simulink model "hps_autopilot_simulink_control_loop"  (R2020a)
settings: Solver=VariableStepAuto  StartTime=0.0  StopTime=10.0  RelTol=1e-3
values from neighbouring files (symbols this model uses):
  Kd = 4    [arduino_matlab.m]
  Ki = 1    [arduino_matlab.m]
  Kp = 1    [arduino_matlab.m]
libraries: checkpacklib x2
settings Model: Creator=ASDFGHJKL  LastModifiedBy=ASDFGHJKL

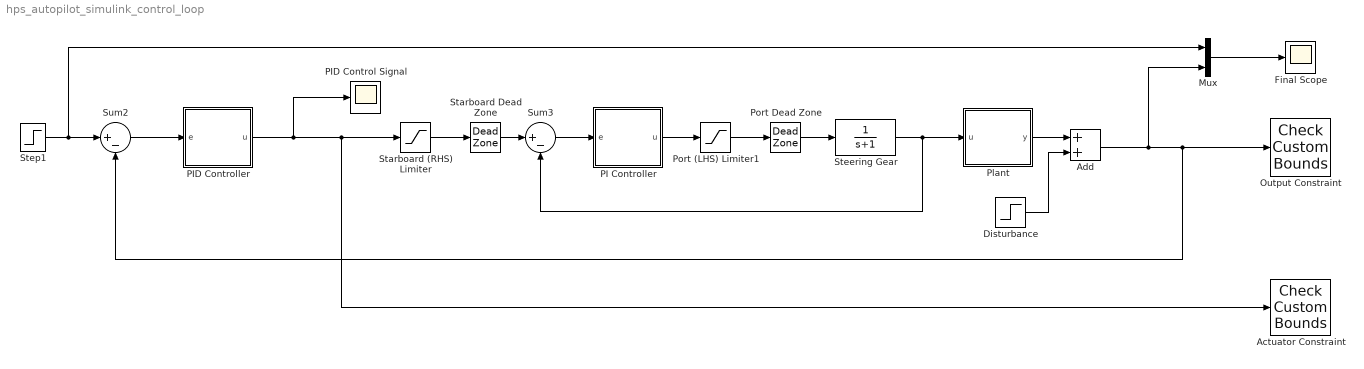
== system hps_autopilot_simulink_control_loop ==
  Actuator Constraint : checkpacklib/Check Custom Bounds  StatePerturbationForJacobian=1.0e-05  InstantiateOnLoad=on  enabled=on  stopWhenAssertionFail=off  export=off  ViewDlgPos=[771.198125 328.725833333334 693.23875 313.738333333334]  OpenViewOnLoad=off  LaunchViewOnOpen=on  TimeUnits=seconds  EnableUpperBound=on  UpperBoundTimes=[0 2.1272365805169;2.1272365805169 20]  UpperBoundAmplitudes=[3.90980563940252 3.90980563940252;0.939113549007046 0.939113549007046]  EnableLowerBound=on  LowerBoundTimes=[0 2.1272365805169;2.1272365805169 20]  LowerBoundAmplitudes=[-3.99363741734438 -3.99363741734438;-0.524055092889176 -0.524055092889176]
      settings: SourceProductBaseCode=CT,ID,MT,SO
  Add : Sum
  Disturbance : Step
  Final Scope : Scope
      settings: StatePerturbationForJacobian=1.0e-05
  Mux : Mux  Inputs=2
  Output Constraint : checkpacklib/Check Custom Bounds  StatePerturbationForJacobian=1.0e-05  InstantiateOnLoad=on  enabled=on  stopWhenAssertionFail=off  export=off  ViewDlgPos=[111.541875 327.726666666666 650.06125 311.74]  OpenViewOnLoad=off  LaunchViewOnOpen=on  TimeUnits=seconds  EnableUpperBound=on  UpperBoundTimes=[0 6;6 20]  UpperBoundAmplitudes=[1.2 1.2;1.01 1.01]  EnableLowerBound=on  LowerBoundTimes=[0 3.2033426183844;3.2033426183844 6;6 20]  LowerBoundAmplitudes=[-0.01 -0.01;0.9 0.9;0.99 0.99]
      settings: SourceProductBaseCode=CT,ID,MT,SO
  PI Controller : Subsystem  StatePerturbationForJacobian=1.0e-05
  PID Control Signal : Scope
  PID Controller : Subsystem  StatePerturbationForJacobian=1.0e-05
  Plant : Subsystem  StatePerturbationForJacobian=1.0e-05
  Port Dead Zone : DeadZone  SaturateOnIntegerOverflow=on
  Port (LHS) Limiter1 : Saturate
  Starboard Dead Zone : DeadZone  SaturateOnIntegerOverflow=on
  Starboard (RHS) Limiter : Saturate
  Steering Gear : TransferFcn  Denominator=[1 1]
  Step1 : Step  StatePerturbationForJacobian=1.0e-05  Time=0.01  SampleTime=0
  Sum2 : Sum  StatePerturbationForJacobian=1.0e-05  Inputs=|+-  SaturateOnIntegerOverflow=on
  Sum3 : Sum  StatePerturbationForJacobian=1.0e-05  Inputs=|+-  SaturateOnIntegerOverflow=on
  wires:
  PI Controller/1(u) -> Port (LHS) Limiter1/1
  PID Controller/1(u) -> Actuator Constraint/1, Starboard (RHS) Limiter/1, PID Control Signal/1
  Disturbance/1 -> Add/2
  Sum3/1 -> PI Controller/1(e)
  Add/1 -> Mux/2, Output Constraint/1, Sum2/2
  Step1/1 -> Mux/1, Sum2/1
  Mux/1 -> Final Scope/1
  Sum2/1 -> PID Controller/1(e)
  Port Dead Zone/1 -> Steering Gear/1
  Steering Gear/1 -> Plant/1("u "), Sum3/2
  Port (LHS) Limiter1/1 -> Port Dead Zone/1
  Plant/1(y) -> Add/1
  Starboard (RHS) Limiter/1 -> Starboard Dead Zone/1
  Starboard Dead Zone/1 -> Sum3/1

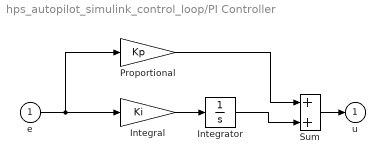
== system hps_autopilot_simulink_control_loop/PI Controller ==
  e : Inport  StatePerturbationForJacobian=1.0e-05
  Integral : Gain  StatePerturbationForJacobian=1.0e-05  Gain=Ki  SaturateOnIntegerOverflow=on  OutDataTypeStr=Inherit: Same as input  ParamDataTypeStr=Inherit: Same as input
  Integrator : Integrator  StatePerturbationForJacobian=1.0e-05
  Proportional : Gain  StatePerturbationForJacobian=1.0e-05  Gain=Kp  SaturateOnIntegerOverflow=on  OutDataTypeStr=Inherit: Same as input  ParamDataTypeStr=Inherit: Same as input
  Sum : Sum  StatePerturbationForJacobian=1.0e-05  InputSameDT=on  SaturateOnIntegerOverflow=on  OutDataTypeStr=Inherit: Same as first input
  u : Outport  StatePerturbationForJacobian=1.0e-05  InitialOutput=0
  wires:
  Proportional/1 -> Sum/1
  Integral/1 -> Integrator/1
  e/1 -> Integral/1, Proportional/1
  Sum/1 -> u/1
  Integrator/1 -> Sum/2

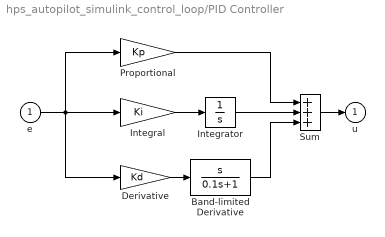
== system hps_autopilot_simulink_control_loop/PID Controller ==
  e : Inport  StatePerturbationForJacobian=1.0e-05
  Band-limited Derivative : TransferFcn  StatePerturbationForJacobian=1.0e-05  Numerator=[1 0]  Denominator=[0.1 1]
  Derivative : Gain  StatePerturbationForJacobian=1.0e-05  Gain=Kd  SaturateOnIntegerOverflow=on  OutDataTypeStr=Inherit: Same as input  ParamDataTypeStr=Inherit: Same as input
  Integral : Gain  StatePerturbationForJacobian=1.0e-05  Gain=Ki  SaturateOnIntegerOverflow=on  OutDataTypeStr=Inherit: Same as input  ParamDataTypeStr=Inherit: Same as input
  Integrator : Integrator  StatePerturbationForJacobian=1.0e-05
  Proportional : Gain  StatePerturbationForJacobian=1.0e-05  Gain=Kp  SaturateOnIntegerOverflow=on  OutDataTypeStr=Inherit: Same as input  ParamDataTypeStr=Inherit: Same as input
  Sum : Sum  StatePerturbationForJacobian=1.0e-05  Inputs=+++  InputSameDT=on  SaturateOnIntegerOverflow=on  OutDataTypeStr=Inherit: Same as first input
  u : Outport  StatePerturbationForJacobian=1.0e-05  InitialOutput=0
  wires:
  Proportional/1 -> Sum/1
  Integral/1 -> Integrator/1
  Band-limited Derivative/1 -> Sum/3
  e/1 -> Integral/1, Proportional/1, Derivative/1
  Sum/1 -> u/1
  Derivative/1 -> Band-limited Derivative/1
  Integrator/1 -> Sum/2

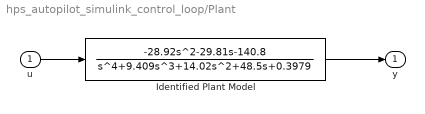
== system hps_autopilot_simulink_control_loop/Plant ==
  "u " : Inport  StatePerturbationForJacobian=1.0e-05
  Identified Plant Model : TransferFcn  StatePerturbationForJacobian=1.0e-05  Numerator=[-28.92 -29.81 -140.8]  Denominator=[1 9.409 14.02 48.5 0.3979]
  y : Outport  StatePerturbationForJacobian=1.0e-05  InitialOutput=0
  wires:
  Identified Plant Model/1 -> y/1
  "u "/1 -> Identified Plant Model/1
